simulink model "SS_Model"  (R2020a)
settings: Solver=VariableStepAuto  StartTime=0.0  StopTime=10  RelTol=1e-3
values from neighbouring files (symbols this model uses):
  A = param{1,1}    [DRL_parameter.m]
  agent = createTD3Agent(numObs,obsInfo,numAct,actInfo,Ts)    [DRL_parameter.m]
  B = param{1,2}    [DRL_parameter.m]
  C = param{1,3}    [DRL_parameter.m]
  D = param{1,4}    [DRL_parameter.m]
  max_Voltage = 10    [DRL_parameter.m]
undefined symbols (not defined in the file or in its folder): getSampleTime
libraries: simulink x3
settings Model: Creator=mohammadim  LastModifiedBy=mohammadim

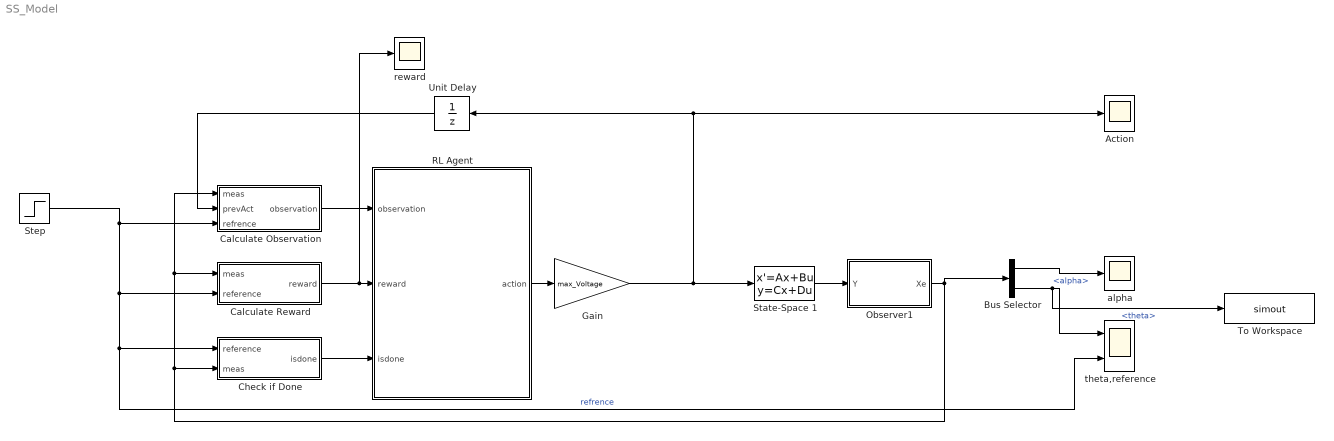
== system SS_Model ==
  Action : Scope
  Bus Selector : BusSelector  OutputSignals=alpha,theta
  Calculate Observation : Subsystem
  Calculate Reward : Subsystem
  Check if Done : Subsystem
  Gain : Gain  Gain=max_Voltage
  Observer1 : Subsystem
  RL Agent : Subsystem  AncestorBlock=rllib/RL Agent  mask(RL Agent){Agent=agent, ProvideReward=on, ProvideIsDone=on, ProvideCumRwd=off, TreatAsDirectFeedthrough=on, CollectLoggedSignals=on, CollectModelStates=on}
      mask prompts: Agent "rl:block:RLAgentAgentPrompt"; ProvideReward "rl:block:RLAgentProvideRewardPrompt"; ProvideIsDone "rl:block:RLAgentProvideIsDonePrompt"; ProvideCumRwd "rl:block:RLAgentProvideCumRwdPrompt"; TreatAsDirectFeedthrough "rl:block:RLAgentDirectFeedthroughPrompt"; CollectLoggedSignals "rl:block:RLAgentCollectLoggedSignalsPrompt"; CollectModelStates "rl:block:RLAgentCollectModelStatesPrompt"
      mask help: rl:block:RLAgentDescription
      mask init:
      | rl.simulink.blocks.agentmaskinit(gcb);
      mask Help: eval('rl.util.guihelp(''rlAgentBlock'')')
      mask DialogControl BDCollapsible Prompt: Block Diagram
      mask DialogControl AgentGroup Prompt: rl:block:RLAgentAgentGroupPrompt
      mask DialogControl Agent Prompt: Agent object
      mask DialogControl Agent Tooltip: rl:block:RLAgentAgentTooltip
      mask DialogControl PortGroup Prompt: rl:block:RLAgentPortsGroupPrompt
      mask DialogControl ProvideReward Prompt: Provide reward signal
      mask DialogControl ProvideReward Tooltip: rl:block:RLAgentProvideRewardTooltip
      mask DialogControl ProvideIsDone Prompt: Provide isdone signal
      mask DialogControl ProvideIsDone Tooltip: rl:block:RLAgentProvideIsDoneTooltip
      mask DialogControl ProvideCumRwd Prompt: Output cumulative reward signal
      mask DialogControl ProvideCumRwd Tooltip: rl:block:RLAgentProvideCumRwdTooltip
      mask DialogControl DirectFeedThroughGroup Prompt: rl:block:RLAgentDirectFeedthroughGroupPrompt
      mask DialogControl TreatAsDirectFeedthrough Prompt: Treat inputs as direct feedthrough
      mask DialogControl TreatAsDirectFeedthrough Tooltip: rl:block:RLAgentDirectFeedthroughTooltip
      mask DialogControl DataGroup Prompt: rl:block:RLAgentDataGroupPrompt
      mask DialogControl CollectLoggedSignals Prompt: Provide logged signals to agent
      mask DialogControl CollectLoggedSignals Tooltip: rl:block:RLAgentCollectLoggedSignalsTooltip
      mask DialogControl CollectModelStates Prompt: Provide model states to agent
      mask DialogControl CollectModelStates Tooltip: rl:block:RLAgentCollectModelStatesTooltip
  State-Space 1 : StateSpace  A=A  B=B  C=C  D=D  InitialCondition=0
  Step : Step  SampleTime=0
  To Workspace : ToWorkspace  VariableName=simout  SaveFormat=Timeseries  SampleTime=-1
  Unit Delay : UnitDelay  SampleTime=-1  HasFrameUpgradeWarning=on
  alpha : Scope
  reward : Scope
  theta,reference : Scope  NumInputPorts=2
  wires:
  Observer1/1(Xe) -> Calculate Reward/1(meas), Calculate Observation/1(meas), Check if Done/2(meas), Bus Selector/1
  State-Space 1/1 -> Observer1/1(Y)
  Check if Done/1(isdone) -> RL Agent/3(isdone)
  Calculate Observation/1(observation) -> RL Agent/1(observation)
  Unit Delay/1 -> Calculate Observation/2(prevAct)
  Calculate Reward/1(reward) -> reward/1, RL Agent/2(reward)
  RL Agent/1(action) -> Gain/1
  Bus Selector/1 -> alpha/1  "<alpha>"
  Bus Selector/2 -> To Workspace/1, theta,reference/1  "<theta>"
  Step/1 -> theta,reference/2, Check if Done/1(reference), Calculate Reward/2(reference), Calculate Observation/3(refrence)  "refrence"
  Gain/1 -> Unit Delay/1, Action/1, State-Space 1/1

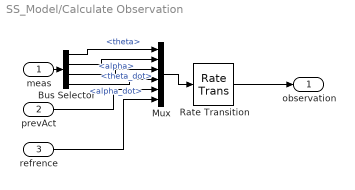
== system SS_Model/Calculate Observation ==
  meas : Inport
  prevAct : Inport  Port=2
  refrence : Inport  Port=3
  Bus Selector : BusSelector  OutputSignals=theta,alpha,theta_dot,alpha_dot
  Mux : Mux  Inputs=6
  Rate Transition : RateTransition
  observation : Outport  VectorParamsAs1DForOutWhenUnconnected=off
  wires:
  prevAct/1 -> Mux/5
  Rate Transition/1 -> observation/1
  Mux/1 -> Rate Transition/1
  meas/1 -> Bus Selector/1
  Bus Selector/1 -> Mux/1  "<theta>"
  Bus Selector/2 -> Mux/2  "<alpha>"
  Bus Selector/3 -> Mux/3  "<theta_dot>"
  Bus Selector/4 -> Mux/4  "<alpha_dot>"
  refrence/1 -> Mux/6

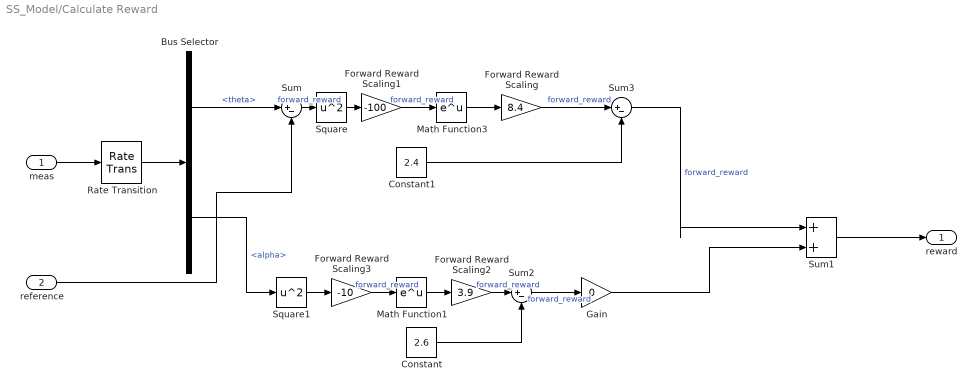
== system SS_Model/Calculate Reward ==
  meas : Inport
  reference : Inport  Port=2
  Bus Selector : BusSelector  OutputSignals=theta,alpha
  Constant : Constant  Value=2.6
  Constant1 : Constant  Value=2.4
  Forward Reward Scaling : Gain  Gain=8.4
  Forward Reward Scaling1 : Gain  Gain=-100
  Forward Reward Scaling2 : Gain  Gain=3.9
  Forward Reward Scaling3 : Gain  Gain=-10
  Gain : Gain  Gain=0
  Math Function1 : Math  SaturateOnIntegerOverflow=on
  Math Function3 : Math  SaturateOnIntegerOverflow=on
  Rate Transition : RateTransition  OutPortSampleTime=Ts
  Square : Math  Operator=square  SaturateOnIntegerOverflow=on
  Square1 : Math  Operator=square  SaturateOnIntegerOverflow=on
  Sum : Sum  Inputs=|+-
  Sum1 : Sum  Inputs=|++
  Sum2 : Sum  Inputs=|+-
  Sum3 : Sum  Inputs=|+-
  reward : Outport  VectorParamsAs1DForOutWhenUnconnected=off
  wires:
  Forward Reward Scaling1/1 -> Math Function3/1  "forward_reward"
  Constant1/1 -> Sum3/2
  Bus Selector/1 -> Sum/1  "<theta>"
  Forward Reward Scaling/1 -> Sum3/1  "forward_reward"
  Square/1 -> Forward Reward Scaling1/1
  meas/1 -> Rate Transition/1
  Math Function3/1 -> Forward Reward Scaling/1
  Sum/1 -> Square/1  "forward_reward"
  Rate Transition/1 -> Bus Selector/1
  reference/1 -> Sum/2
  Math Function1/1 -> Forward Reward Scaling2/1
  Bus Selector/2 -> Square1/1  "<alpha>"
  Forward Reward Scaling3/1 -> Math Function1/1  "forward_reward"
  Forward Reward Scaling2/1 -> Sum2/1  "forward_reward"
  Square1/1 -> Forward Reward Scaling3/1
  Constant/1 -> Sum2/2
  Sum1/1 -> reward/1
  Sum3/1 -> Sum1/1  "forward_reward"
  Sum2/1 -> Gain/1  "forward_reward"
  Gain/1 -> Sum1/2

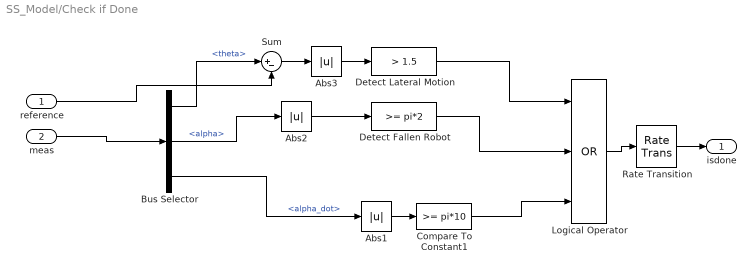
== system SS_Model/Check if Done ==
  reference : Inport
  meas : Inport  Port=2
  Abs1 : Abs
  Abs2 : Abs
  Abs3 : Abs
  Bus Selector : BusSelector  OutputSignals=theta,alpha,alpha_dot
  Compare To Constant1 : simulink/Logic and Bit Operations/Compare To Constant  relop=>=  const=pi*10  OutDataTypeStr=boolean
  Detect Fallen Robot : simulink/Logic and Bit Operations/Compare To Constant  relop=>=  const=pi*2  OutDataTypeStr=boolean
  Detect Lateral Motion : simulink/Logic and Bit Operations/Compare To Constant  relop=>  const=1.5  OutDataTypeStr=boolean
  Logical Operator : Logic  Operator=OR  Inputs=3  AllPortsSameDT=off  OutDataTypeStr=boolean
  Rate Transition : RateTransition
  Sum : Sum  Inputs=|+-
  isdone : Outport  VectorParamsAs1DForOutWhenUnconnected=off
  wires:
  Detect Lateral Motion/1 -> Logical Operator/1
  Abs3/1 -> Detect Lateral Motion/1
  Rate Transition/1 -> isdone/1
  Compare To Constant1/1 -> Logical Operator/3
  Abs1/1 -> Compare To Constant1/1
  Bus Selector/3 -> Abs1/1  "<alpha_dot>"
  Detect Fallen Robot/1 -> Logical Operator/2
  Logical Operator/1 -> Rate Transition/1
  meas/1 -> Bus Selector/1
  Abs2/1 -> Detect Fallen Robot/1
  Bus Selector/2 -> Abs2/1  "<alpha>"
  Bus Selector/1 -> Sum/1  "<theta>"
  Sum/1 -> Abs3/1
  reference/1 -> Sum/2

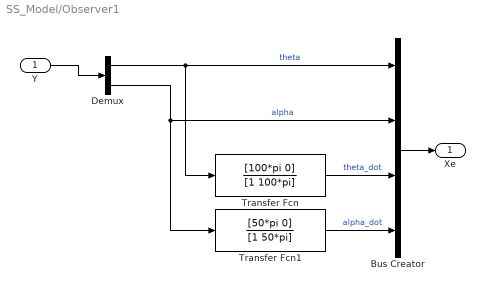
== system SS_Model/Observer1 ==
  Y : Inport
  Bus Creator : BusCreator  Inputs=4
  Demux : Demux  Outputs=2
  Transfer Fcn : TransferFcn  Numerator=[100*pi 0]  Denominator=[1 100*pi]
  Transfer Fcn1 : TransferFcn  Numerator=[50*pi 0]  Denominator=[1 50*pi]
  Xe : Outport
  wires:
  Transfer Fcn1/1 -> Bus Creator/4  "alpha_dot"
  Demux/1 -> Transfer Fcn/1, Bus Creator/1  "theta"
  Transfer Fcn/1 -> Bus Creator/3  "theta_dot"
  Y/1 -> Demux/1
  Bus Creator/1 -> Xe/1
  Demux/2 -> Transfer Fcn1/1, Bus Creator/2  "alpha"

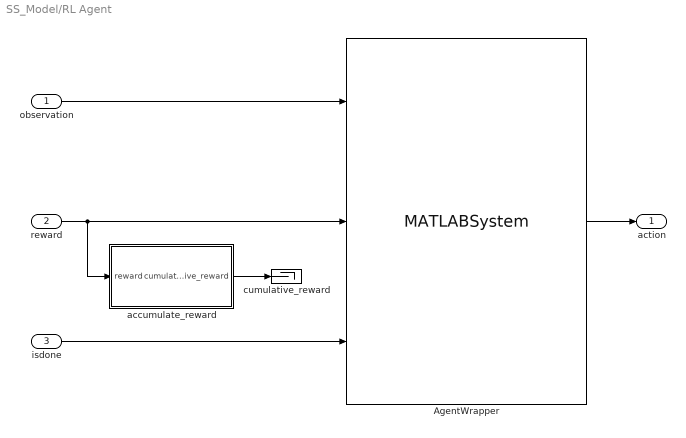
== system SS_Model/RL Agent ==
  observation : Inport
  reward : Inport  Port=2
  isdone : Inport  Port=3
  AgentWrapper : MATLABSystem  System=rl.simulink.blocks.AgentWrapper  ModelName=SS_Model  AgentObjectName=Agent  BlockPath=SS_Model/RL Agent/AgentWrapper  TreatAsDirectFeedthrough=true  IsRewardProvided=true  IsIsDoneProvided=true  CollectLoggedSignals=true  CollectModelStates=true
      mask Type: rl.simulink.blocks.AgentWrapper
      mask Display:
      | disp('AgentWrapper');
      | port_label('input',1,'observation');
      | port_label('input',2,'reward');
      | port_label('input',3,'isdone');
      | port_label('output',1,'action');
  accumulate_reward : Subsystem
  cumulative_reward : Terminator
  action : Outport  VectorParamsAs1DForOutWhenUnconnected=off
  wires:
  accumulate_reward/1(cumulative_reward) -> cumulative_reward/1
  isdone/1 -> AgentWrapper/3
  reward/1 -> AgentWrapper/2, accumulate_reward/1(reward)
  AgentWrapper/1 -> action/1
  observation/1 -> AgentWrapper/1

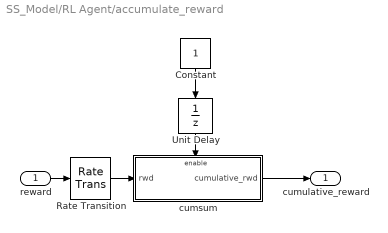
== system SS_Model/RL Agent/accumulate_reward ==
  reward : Inport
  Constant : Constant
  Rate Transition : RateTransition  OutPortSampleTime=getSampleTime(Agent)
  Unit Delay : UnitDelay  SampleTime=-1  HasFrameUpgradeWarning=on
  cumsum : Subsystem
  cumulative_reward : Outport  VectorParamsAs1DForOutWhenUnconnected=off
  wires:
  Rate Transition/1 -> cumsum/1(rwd)
  reward/1 -> Rate Transition/1
  Constant/1 -> Unit Delay/1
  Unit Delay/1 -> cumsum/Enable
  cumsum/1(cumulative_rwd) -> cumulative_reward/1

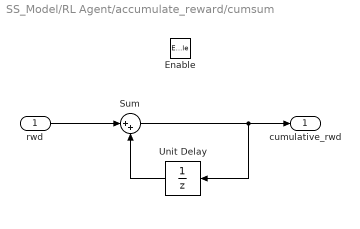
== system SS_Model/RL Agent/accumulate_reward/cumsum ==
  rwd : Inport
  Enable : EnablePort
  Sum : Sum  Inputs=|++
  Unit Delay : UnitDelay  SampleTime=-1  HasFrameUpgradeWarning=on
  cumulative_rwd : Outport  VectorParamsAs1DForOutWhenUnconnected=off
  wires:
  Unit Delay/1 -> Sum/2
  Sum/1 -> cumulative_rwd/1, Unit Delay/1
  rwd/1 -> Sum/1
